simulink model "simu_main"  (R2025b)
settings: Solver=ode5  StartTime=0.0  StopTime=50  RelTol=1e-3
StartFcn:
  | MaxMissedTicks = 99^100;
  | SampleTime = 0.01;
undefined symbols (not defined in the file or in its folder): National_Instruments, PCI
libraries: sldrtlib x6
settings Model: Creator=labadmin  LastModifiedBy=aie4-26
settings HardwareCC: ProdBitPerLong=64.0  ProdHWDeviceType=Intel->x86-64 (Linux 64)
settings RTWCC: SystemTargetFile=sldrt.tlc  TemplateMakefile=sldrt.tmf  RTWCompilerOptimization=on  GPUComputeCapability=3.5  Description=Simulink Desktop Real-Time
settings CodeAppCC: MaxIdLength=95.0
settings SimulinkDesktopRealTimeCC: ExtModeTransport=0.0  ExtModeStaticAllocSize=1000000.0  TargetLibSuffix=_sldrt.a  TargetPreCompLibLocation=C:\Program Files\MATLAB\R2025b\toolbox\sldrt\lib\win64  MultiwordLength=2048.0  DynamicStringBufferSize=256.0  ParMdlRefBuildCompliant=on  PreserveMATLABNamespacesInGeneratedCode=on  SubcomponentCodeInterfacePackaging=Reusable function

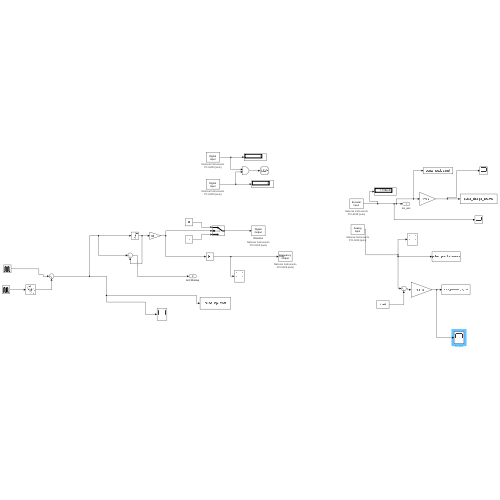
[thumbnail: Simulink's stored preview of the top-level diagram]
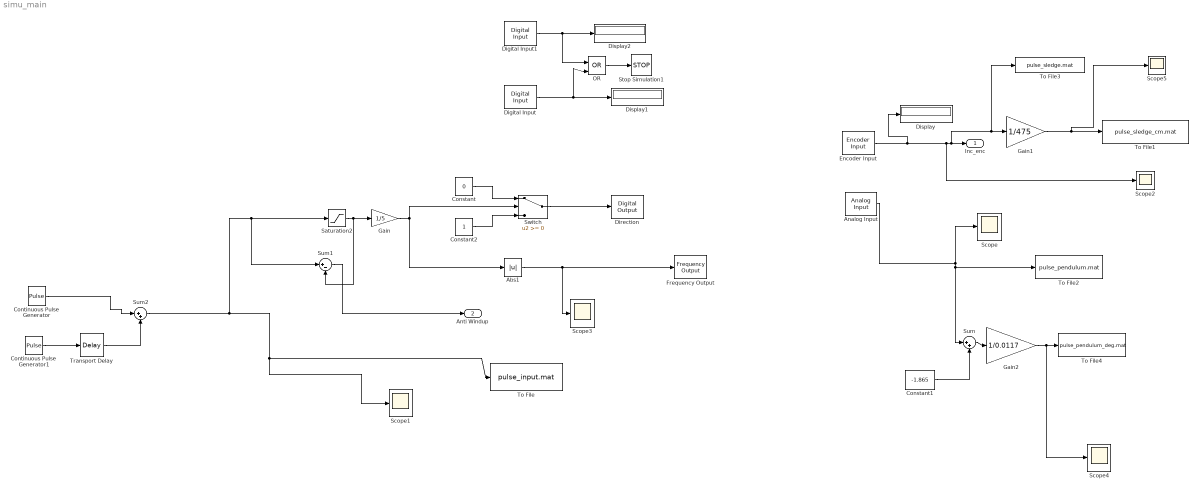
== system simu_main ==
  Abs1 : Abs  SaturateOnIntegerOverflow=off
  Analog Input : sldrtlib/Analog Input  SampleTime=SampleTime  MaxMissedTicks=MaxMissedTicks  ShowMissedTicks=off  YieldWhenWaiting=off  DrvName=National_Instruments/PCI-6229  DrvAddress=4294967295  DrvOptions=[1 1 8192 2 3]  Channels=1  RangeMode=1  VoltRange=1  DataType=1
      settings: AttributesFormatString=National Instruments\nPCI-6229 [auto]
  Constant : Constant  Value=0  SampleTime=SampleTime
  Constant1 : Constant  Value=-1.865
  Constant2 : Constant  SampleTime=SampleTime
  Continuous Pulse Generator : DiscretePulseGenerator  PulseType=Time based  Amplitude=1.8  Period=20  PulseWidth=5
  Continuous Pulse Generator1 : DiscretePulseGenerator  PulseType=Time based  Amplitude=-1.8  Period=20  PulseWidth=5
  Digital Input : sldrtlib/Digital Input  SampleTime=0.1  MaxMissedTicks=10  ShowMissedTicks=off  YieldWhenWaiting=off  DrvName=National_Instruments/PCI-6229  DrvAddress=4294967295  DrvOptions=[1 1 8192 2 3]  Channels=2  BitMode=1  DataType=1
      settings: AttributesFormatString=National Instruments\nPCI-6229 [auto]
  Digital Input1 : sldrtlib/Digital Input  SampleTime=0.1  MaxMissedTicks=10  ShowMissedTicks=off  YieldWhenWaiting=off  DrvName=National_Instruments/PCI-6229  DrvAddress=4294967295  DrvOptions=[1 1 8192 2 3]  Channels=3  BitMode=1  DataType=9
      settings: AttributesFormatString=National Instruments\nPCI-6229 [auto]
  Direction : sldrtlib/Digital Output  SampleTime=SampleTime  MaxMissedTicks=MaxMissedTicks  ShowMissedTicks=off  YieldWhenWaiting=off  DrvName=National_Instruments/PCI-6229  DrvAddress=4294967295  DrvOptions=[1 1 8192 2 3]  Channels=1  BitMode=1  InitialValue=0  FinalValue=0
      settings: AttributesFormatString=National Instruments\nPCI-6229 [auto]
  Display : Display
  Display1 : Display
  Display2 : Display
  Encoder Input : sldrtlib/Encoder Input  SampleTime=SampleTime  MaxMissedTicks=MaxMissedTicks  ShowMissedTicks=off  YieldWhenWaiting=off  DrvName=National_Instruments/PCI-6229  DrvAddress=4294967295  DrvOptions=[1 1 8192 2 3]  Channels=1  QuadMode=3  IndexPulse=2  InputFilter=Inf  DataType=1
      settings: AttributesFormatString=National Instruments\nPCI-6229 [auto]
  Frequency Output : sldrtlib/Frequency Output  SampleTime=SampleTime  MaxMissedTicks=MaxMissedTicks  ShowMissedTicks=off  YieldWhenWaiting=off  DrvName=National_Instruments/PCI-6229  DrvAddress=4294967295  DrvOptions=[1 1 8192 2 3]  Channels=2  FrequencySource=1  Frequency=10000  FrequencyFinalValue=[]  DutySource=2  Duty=0  DutyFinalValue=0
      settings: AttributesFormatString=National Instruments\nPCI-6229 [auto]
  Gain : Gain  Gain=1/5
  Gain1 : Gain  Gain=1/475
  Gain2 : Gain  Gain=1/0.0117
  OR : Logic  Operator=OR  IconShape=distinctive  AllPortsSameDT=off  OutDataTypeStr=boolean
  Saturation2 : Saturate  UpperLimit=2.5  LowerLimit=-2.5
  Scope{,1..5} (6 alike) : Scope
      Scope settings: ActiveDisplayYMinimum=1.12811121131901  ActiveDisplayYMaximum=2.5477596350743013
      Scope1 settings: ActiveDisplayYMinimum=-2.2499999389130094  ActiveDisplayYMaximum=2.2499997060145476
      Scope2 settings: ActiveDisplayYMinimum=-6365.75  ActiveDisplayYMaximum=8181.75  DataLoggingVariableName=ScopeData2
      Scope3 settings: ActiveDisplayYMinimum=-0.0026912727390916436  ActiveDisplayYMaximum=0.51518028613937739  DataLoggingVariableName=ScopeData3
      Scope4 settings: ActiveDisplayYMinimum=-32.287261610322055  ActiveDisplayYMaximum=31.014728470615673  DataLoggingVariableName=ScopeData4
      Scope5 settings: ActiveDisplayYMinimum=-40.941052631578948  ActiveDisplayYMaximum=55.732631578947363  DataLoggingVariableName=ScopeData5
  Stop Simulation1 : Stop
  Sum : Sum  Inputs=|++
  Sum1 : Sum  Inputs=|+-
  Sum2 : Sum  Inputs=|++
  Switch : Switch  SaturateOnIntegerOverflow=off  InputSameDT=off
  To File : ToFile  Filename=pulse_input.mat  SaveFormat=Timeseries
  To File1 : ToFile  Filename=pulse_sledge_cm.mat  SaveFormat=Timeseries
  To File2 : ToFile  Filename=pulse_pendulum.mat  SaveFormat=Timeseries
  To File3 : ToFile  Filename=pulse_sledge.mat  SaveFormat=Timeseries
  To File4 : ToFile  Filename=pulse_pendulum_deg.mat  SaveFormat=Timeseries
  Transport Delay : TransportDelay  DelayTime=10
  Inc_enc : Outport
  Anti Windup : Outport  Port=2
  wires:
  Sum1/1 -> Anti Windup/1
  Switch/1 -> Direction/1
  Gain/1 -> Abs1/1, Switch/2
  Saturation2/1 -> Sum1/2, Gain/1
  Constant2/1 -> Switch/3
  Encoder Input/1 -> Display/1, Scope2/1, To File3/1, Gain1/1, Inc_enc/1
  Constant/1 -> Switch/1
  Digital Input/1 -> OR/2, Display1/1
  Digital Input1/1 -> OR/1, Display2/1
  Abs1/1 -> Scope3/1, Frequency Output/1
  OR/1 -> Stop Simulation1/1
  Analog Input/1 -> Sum/1, To File2/1, Scope/1
  Gain1/1 -> Scope5/1, To File1/1
  Gain2/1 -> Scope4/1, To File4/1
  Sum/1 -> Gain2/1
  Constant1/1 -> Sum/2
  Sum2/1 -> Saturation2/1, Sum1/1, Scope1/1, To File/1
  Continuous Pulse Generator1/1 -> Transport Delay/1
  Continuous Pulse Generator/1 -> Sum2/1
  Transport Delay/1 -> Sum2/2
